simulink model "untitled1"  (R2022a)
settings: Solver=VariableStepAuto  StartTime=0.0  StopTime=10.0  RelTol=1e-3
undefined symbols (not defined in the file or in its folder): D, J_i, J_m, K_e, K_t, L, R
settings Model: Creator=Hoshi Kairi  LastModifiedBy=Hoshi Kairi

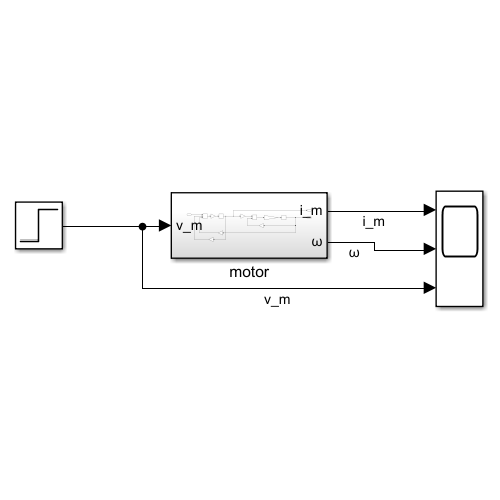
[thumbnail: Simulink's stored preview of the top-level diagram]
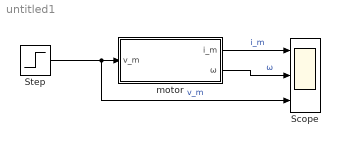
== system untitled1 ==
  Scope : Scope  NumInputPorts=3
  Step : Step  SampleTime=0
  motor : Subsystem
  wires:
  Step/1 -> Scope/3, motor/1(v_m)  "v_m"
  motor/1(i_m) -> Scope/1  "i_m"
  motor/2(ω) -> Scope/2  "ω"

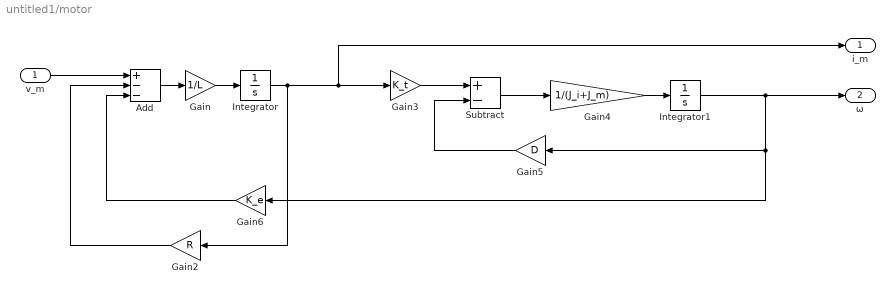
== system untitled1/motor ==
  v_m : Inport
  Add : Sum  Inputs=+--
  Gain : Gain  Gain=1/L
  Gain2 : Gain  Gain=R
  Gain3 : Gain  Gain=K_t
  Gain4 : Gain  Gain=1/(J_i+J_m)
  Gain5 : Gain  Gain=D
  Gain6 : Gain  Gain=K_e
  Integrator : Integrator
  Integrator1 : Integrator
  Subtract : Sum  Inputs=+-
  i_m : Outport
  ω : Outport  Port=2
  wires:
  v_m/1 -> Add/1
  Add/1 -> Gain/1
  Gain/1 -> Integrator/1
  Integrator/1 -> i_m/1, Gain3/1, Gain2/1
  Gain2/1 -> Add/2
  Gain3/1 -> Subtract/1
  Gain4/1 -> Integrator1/1
  Integrator1/1 -> Gain6/1, Gain5/1, ω/1
  Gain5/1 -> Subtract/2
  Gain6/1 -> Add/3
  Subtract/1 -> Gain4/1
